simulink model "Sim7"  (R2021b)
settings: Solver=FixedStepDiscrete  StartTime=0.0  StopTime=1  FixedStep=1e-6  RelTol=1e-3  EnableMultiTasking=on
InitFcn:
  | clc
  | Ts=1e-6;
  | ts=Ts;
  | Td=Ts;
  | disp(sprintf('Ts = %f',Ts))
  |  %1/fs = sampling period;
  | Ts = Td;
  | Tch = Td;
  | 
  | %harmonics
  | kh=0;
  | 
  | % PLL
  | Tset = 0.1; % settling time
  | zeta = 0.707;   % damping ratio (optimized for best response of the second order TF
  | 
  | %grid params
  | tha = 0;
  | kh = 0;
  | V1 = 230;
  | fg = 50;
  | 
  | %freq var
  | onoff = 0;
  | onoff_faults = 1;
  | fperiod = 2;
  | fmin = 48;
  | fmax = 52;
undefined symbols (not defined in the file or in its folder): DiscIntNeverNeededParam
libraries: spsThreePhaseSeriesRLCBranchLib x8, powerlib_extras x5, spsThreePhaseVIMeasurementLib x5, spsSeriesRLCBranchLib x3, spsUniversalBridgeLib x3, spsGroundLib x2, spsDCVoltageSourceLib x2, spsThreePhaseBreakerLib x2, spspowerguiLib x1
(part 2 of 2)

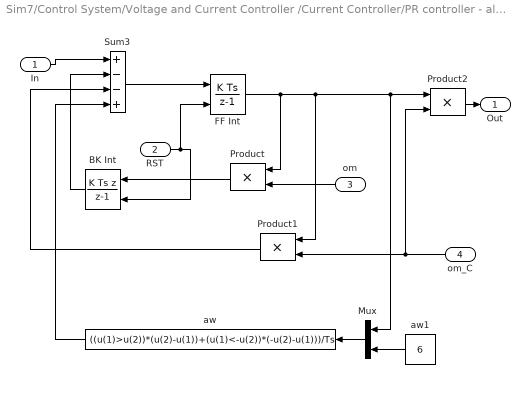
== system Sim7/Control System/Voltage and Current Controller /Current Controller/PR controller - alpha/RES1 ==
  In : Inport
  RST : Inport  Port=2
  om : Inport  Port=3
  om_C : Inport  Port=4
  BK Int : DiscreteIntegrator  IntegratorMethod=Integration: Backward Euler  ExternalReset=level  InitialCondition=-100000  SampleTime=-1  ICPrevOutput=DiscIntNeverNeededParam  ICPrevScaledInput=DiscIntNeverNeededParam
  FF Int : DiscreteIntegrator  ExternalReset=level  SampleTime=-1  ICPrevOutput=DiscIntNeverNeededParam  ICPrevScaledInput=DiscIntNeverNeededParam
  Mux : Mux  Inputs=2
  Product : Product  SaturateOnIntegerOverflow=on  OutDataTypeStr=Inherit: Same as first input
  Product1 : Product  SaturateOnIntegerOverflow=on  OutDataTypeStr=Inherit: Same as first input
  Product2 : Product  SaturateOnIntegerOverflow=on  OutDataTypeStr=Inherit: Same as first input
  Sum3 : Sum  Inputs=+--+  SaturateOnIntegerOverflow=on
  aw : Fcn  Expr=((u(1)>u(2))*(u(2)-u(1))+(u(1)<-u(2))*(-u(2)-u(1)))/Ts
  aw1 : Constant  Value=6
  Out : Outport
  wires:
  om/1 -> Product/2
  aw1/1 -> Mux/2
  Mux/1 -> aw/1
  RST/1 -> FF Int/2, BK Int/2
  BK Int/1 -> Sum3/2
  FF Int/1 -> Product/1, Product1/1, Mux/1, Product2/1
  Product/1 -> BK Int/1
  In/1 -> Sum3/1
  om_C/1 -> Product1/2, Product2/2
  aw/1 -> Sum3/4
  Product1/1 -> Sum3/3
  Sum3/1 -> FF Int/1
  Product2/1 -> Out/1

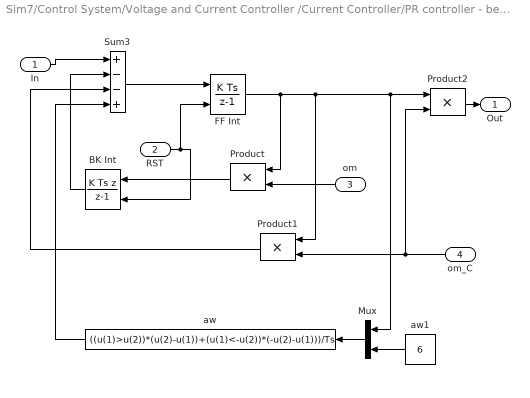
== system Sim7/Control System/Voltage and Current Controller /Current Controller/PR controller - beta/RES1 ==
  In : Inport
  RST : Inport  Port=2
  om : Inport  Port=3
  om_C : Inport  Port=4
  BK Int : DiscreteIntegrator  IntegratorMethod=Integration: Backward Euler  ExternalReset=level  InitialCondition=-100000  SampleTime=-1  ICPrevOutput=DiscIntNeverNeededParam  ICPrevScaledInput=DiscIntNeverNeededParam
  FF Int : DiscreteIntegrator  ExternalReset=level  SampleTime=-1  ICPrevOutput=DiscIntNeverNeededParam  ICPrevScaledInput=DiscIntNeverNeededParam
  Mux : Mux  Inputs=2
  Product : Product  SaturateOnIntegerOverflow=on  OutDataTypeStr=Inherit: Same as first input
  Product1 : Product  SaturateOnIntegerOverflow=on  OutDataTypeStr=Inherit: Same as first input
  Product2 : Product  SaturateOnIntegerOverflow=on  OutDataTypeStr=Inherit: Same as first input
  Sum3 : Sum  Inputs=+--+  SaturateOnIntegerOverflow=on
  aw : Fcn  Expr=((u(1)>u(2))*(u(2)-u(1))+(u(1)<-u(2))*(-u(2)-u(1)))/Ts
  aw1 : Constant  Value=6
  Out : Outport
  wires:
  om/1 -> Product/2
  aw1/1 -> Mux/2
  Mux/1 -> aw/1
  RST/1 -> FF Int/2, BK Int/2
  BK Int/1 -> Sum3/2
  FF Int/1 -> Product/1, Product1/1, Mux/1, Product2/1
  Product/1 -> BK Int/1
  In/1 -> Sum3/1
  om_C/1 -> Product1/2, Product2/2
  aw/1 -> Sum3/4
  Product1/1 -> Sum3/3
  Sum3/1 -> FF Int/1
  Product2/1 -> Out/1

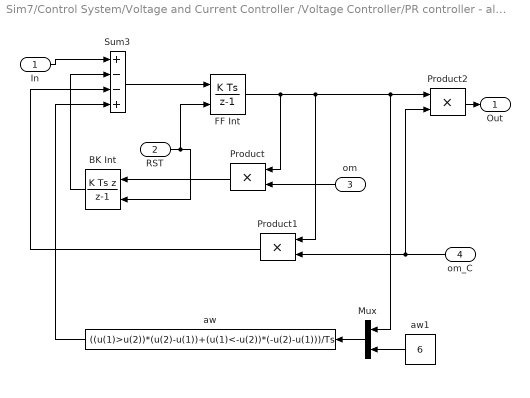
== system Sim7/Control System/Voltage and Current Controller /Voltage Controller/PR controller - alpha/RES1 ==
  In : Inport
  RST : Inport  Port=2
  om : Inport  Port=3
  om_C : Inport  Port=4
  BK Int : DiscreteIntegrator  IntegratorMethod=Integration: Backward Euler  ExternalReset=level  InitialCondition=-100000  SampleTime=-1  ICPrevOutput=DiscIntNeverNeededParam  ICPrevScaledInput=DiscIntNeverNeededParam
  FF Int : DiscreteIntegrator  ExternalReset=level  SampleTime=-1  ICPrevOutput=DiscIntNeverNeededParam  ICPrevScaledInput=DiscIntNeverNeededParam
  Mux : Mux  Inputs=2
  Product : Product  SaturateOnIntegerOverflow=on  OutDataTypeStr=Inherit: Same as first input
  Product1 : Product  SaturateOnIntegerOverflow=on  OutDataTypeStr=Inherit: Same as first input
  Product2 : Product  SaturateOnIntegerOverflow=on  OutDataTypeStr=Inherit: Same as first input
  Sum3 : Sum  Inputs=+--+  SaturateOnIntegerOverflow=on
  aw : Fcn  Expr=((u(1)>u(2))*(u(2)-u(1))+(u(1)<-u(2))*(-u(2)-u(1)))/Ts
  aw1 : Constant  Value=6
  Out : Outport
  wires:
  om/1 -> Product/2
  aw1/1 -> Mux/2
  Mux/1 -> aw/1
  RST/1 -> FF Int/2, BK Int/2
  BK Int/1 -> Sum3/2
  FF Int/1 -> Product/1, Product1/1, Mux/1, Product2/1
  Product/1 -> BK Int/1
  In/1 -> Sum3/1
  om_C/1 -> Product1/2, Product2/2
  aw/1 -> Sum3/4
  Product1/1 -> Sum3/3
  Sum3/1 -> FF Int/1
  Product2/1 -> Out/1

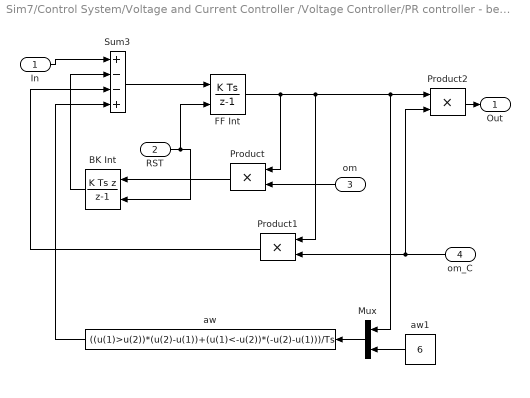
== system Sim7/Control System/Voltage and Current Controller /Voltage Controller/PR controller - beta/RES1 ==
  In : Inport
  RST : Inport  Port=2
  om : Inport  Port=3
  om_C : Inport  Port=4
  BK Int : DiscreteIntegrator  IntegratorMethod=Integration: Backward Euler  ExternalReset=level  InitialCondition=-100000  SampleTime=-1  ICPrevOutput=DiscIntNeverNeededParam  ICPrevScaledInput=DiscIntNeverNeededParam
  FF Int : DiscreteIntegrator  ExternalReset=level  SampleTime=-1  ICPrevOutput=DiscIntNeverNeededParam  ICPrevScaledInput=DiscIntNeverNeededParam
  Mux : Mux  Inputs=2
  Product : Product  SaturateOnIntegerOverflow=on  OutDataTypeStr=Inherit: Same as first input
  Product1 : Product  SaturateOnIntegerOverflow=on  OutDataTypeStr=Inherit: Same as first input
  Product2 : Product  SaturateOnIntegerOverflow=on  OutDataTypeStr=Inherit: Same as first input
  Sum3 : Sum  Inputs=+--+  SaturateOnIntegerOverflow=on
  aw : Fcn  Expr=((u(1)>u(2))*(u(2)-u(1))+(u(1)<-u(2))*(-u(2)-u(1)))/Ts
  aw1 : Constant  Value=6
  Out : Outport
  wires:
  om/1 -> Product/2
  aw1/1 -> Mux/2
  Mux/1 -> aw/1
  RST/1 -> FF Int/2, BK Int/2
  BK Int/1 -> Sum3/2
  FF Int/1 -> Product/1, Product1/1, Mux/1, Product2/1
  Product/1 -> BK Int/1
  In/1 -> Sum3/1
  om_C/1 -> Product1/2, Product2/2
  aw/1 -> Sum3/4
  Product1/1 -> Sum3/3
  Sum3/1 -> FF Int/1
  Product2/1 -> Out/1

== system Sim7/Control System2/Voltage and Current Controller/Current Controller/PR controller - alpha/RES1 ==
  In : Inport
  RST : Inport  Port=2
  om : Inport  Port=3
  om_C : Inport  Port=4
  BK Int : DiscreteIntegrator  IntegratorMethod=Integration: Backward Euler  ExternalReset=level  InitialCondition=-100000  SampleTime=-1  ICPrevOutput=DiscIntNeverNeededParam  ICPrevScaledInput=DiscIntNeverNeededParam
  FF Int : DiscreteIntegrator  ExternalReset=level  SampleTime=-1  ICPrevOutput=DiscIntNeverNeededParam  ICPrevScaledInput=DiscIntNeverNeededParam
  Mux : Mux  Inputs=2
  Product : Product  SaturateOnIntegerOverflow=on  OutDataTypeStr=Inherit: Same as first input
  Product1 : Product  SaturateOnIntegerOverflow=on  OutDataTypeStr=Inherit: Same as first input
  Product2 : Product  SaturateOnIntegerOverflow=on  OutDataTypeStr=Inherit: Same as first input
  Sum3 : Sum  Inputs=+--+  SaturateOnIntegerOverflow=on
  aw : Fcn  Expr=((u(1)>u(2))*(u(2)-u(1))+(u(1)<-u(2))*(-u(2)-u(1)))/Ts
  aw1 : Constant  Value=6
  Out : Outport
  wires:
  om/1 -> Product/2
  aw1/1 -> Mux/2
  Mux/1 -> aw/1
  RST/1 -> FF Int/2, BK Int/2
  BK Int/1 -> Sum3/2
  FF Int/1 -> Product/1, Product1/1, Mux/1, Product2/1
  Product/1 -> BK Int/1
  In/1 -> Sum3/1
  om_C/1 -> Product1/2, Product2/2
  aw/1 -> Sum3/4
  Product1/1 -> Sum3/3
  Sum3/1 -> FF Int/1
  Product2/1 -> Out/1

== system Sim7/Control System2/Voltage and Current Controller/Current Controller/PR controller - beta/RES1 ==
  In : Inport
  RST : Inport  Port=2
  om : Inport  Port=3
  om_C : Inport  Port=4
  BK Int : DiscreteIntegrator  IntegratorMethod=Integration: Backward Euler  ExternalReset=level  InitialCondition=-100000  SampleTime=-1  ICPrevOutput=DiscIntNeverNeededParam  ICPrevScaledInput=DiscIntNeverNeededParam
  FF Int : DiscreteIntegrator  ExternalReset=level  SampleTime=-1  ICPrevOutput=DiscIntNeverNeededParam  ICPrevScaledInput=DiscIntNeverNeededParam
  Mux : Mux  Inputs=2
  Product : Product  SaturateOnIntegerOverflow=on  OutDataTypeStr=Inherit: Same as first input
  Product1 : Product  SaturateOnIntegerOverflow=on  OutDataTypeStr=Inherit: Same as first input
  Product2 : Product  SaturateOnIntegerOverflow=on  OutDataTypeStr=Inherit: Same as first input
  Sum3 : Sum  Inputs=+--+  SaturateOnIntegerOverflow=on
  aw : Fcn  Expr=((u(1)>u(2))*(u(2)-u(1))+(u(1)<-u(2))*(-u(2)-u(1)))/Ts
  aw1 : Constant  Value=6
  Out : Outport
  wires:
  om/1 -> Product/2
  aw1/1 -> Mux/2
  Mux/1 -> aw/1
  RST/1 -> FF Int/2, BK Int/2
  BK Int/1 -> Sum3/2
  FF Int/1 -> Product/1, Product1/1, Mux/1, Product2/1
  Product/1 -> BK Int/1
  In/1 -> Sum3/1
  om_C/1 -> Product1/2, Product2/2
  aw/1 -> Sum3/4
  Product1/1 -> Sum3/3
  Sum3/1 -> FF Int/1
  Product2/1 -> Out/1

== system Sim7/Control System2/Voltage and Current Controller/Voltage Controller/PR controller - alpha/RES1 ==
  In : Inport
  RST : Inport  Port=2
  om : Inport  Port=3
  om_C : Inport  Port=4
  BK Int : DiscreteIntegrator  IntegratorMethod=Integration: Backward Euler  ExternalReset=level  InitialCondition=-100000  SampleTime=-1  ICPrevOutput=DiscIntNeverNeededParam  ICPrevScaledInput=DiscIntNeverNeededParam
  FF Int : DiscreteIntegrator  ExternalReset=level  SampleTime=-1  ICPrevOutput=DiscIntNeverNeededParam  ICPrevScaledInput=DiscIntNeverNeededParam
  Mux : Mux  Inputs=2
  Product : Product  SaturateOnIntegerOverflow=on  OutDataTypeStr=Inherit: Same as first input
  Product1 : Product  SaturateOnIntegerOverflow=on  OutDataTypeStr=Inherit: Same as first input
  Product2 : Product  SaturateOnIntegerOverflow=on  OutDataTypeStr=Inherit: Same as first input
  Sum3 : Sum  Inputs=+--+  SaturateOnIntegerOverflow=on
  aw : Fcn  Expr=((u(1)>u(2))*(u(2)-u(1))+(u(1)<-u(2))*(-u(2)-u(1)))/Ts
  aw1 : Constant  Value=6
  Out : Outport
  wires:
  om/1 -> Product/2
  aw1/1 -> Mux/2
  Mux/1 -> aw/1
  RST/1 -> FF Int/2, BK Int/2
  BK Int/1 -> Sum3/2
  FF Int/1 -> Product/1, Product1/1, Mux/1, Product2/1
  Product/1 -> BK Int/1
  In/1 -> Sum3/1
  om_C/1 -> Product1/2, Product2/2
  aw/1 -> Sum3/4
  Product1/1 -> Sum3/3
  Sum3/1 -> FF Int/1
  Product2/1 -> Out/1

== system Sim7/Control System2/Voltage and Current Controller/Voltage Controller/PR controller - beta/RES1 ==
  In : Inport
  RST : Inport  Port=2
  om : Inport  Port=3
  om_C : Inport  Port=4
  BK Int : DiscreteIntegrator  IntegratorMethod=Integration: Backward Euler  ExternalReset=level  InitialCondition=-100000  SampleTime=-1  ICPrevOutput=DiscIntNeverNeededParam  ICPrevScaledInput=DiscIntNeverNeededParam
  FF Int : DiscreteIntegrator  ExternalReset=level  SampleTime=-1  ICPrevOutput=DiscIntNeverNeededParam  ICPrevScaledInput=DiscIntNeverNeededParam
  Mux : Mux  Inputs=2
  Product : Product  SaturateOnIntegerOverflow=on  OutDataTypeStr=Inherit: Same as first input
  Product1 : Product  SaturateOnIntegerOverflow=on  OutDataTypeStr=Inherit: Same as first input
  Product2 : Product  SaturateOnIntegerOverflow=on  OutDataTypeStr=Inherit: Same as first input
  Sum3 : Sum  Inputs=+--+  SaturateOnIntegerOverflow=on
  aw : Fcn  Expr=((u(1)>u(2))*(u(2)-u(1))+(u(1)<-u(2))*(-u(2)-u(1)))/Ts
  aw1 : Constant  Value=6
  Out : Outport
  wires:
  om/1 -> Product/2
  aw1/1 -> Mux/2
  Mux/1 -> aw/1
  RST/1 -> FF Int/2, BK Int/2
  BK Int/1 -> Sum3/2
  FF Int/1 -> Product/1, Product1/1, Mux/1, Product2/1
  Product/1 -> BK Int/1
  In/1 -> Sum3/1
  om_C/1 -> Product1/2, Product2/2
  aw/1 -> Sum3/4
  Product1/1 -> Sum3/3
  Sum3/1 -> FF Int/1
  Product2/1 -> Out/1
